simulink model "simulation_diffeomorfisme"  (R2020a)
settings: Solver=VariableStepAuto  StartTime=0.0  StopTime=100  RelTol=1e-3
values from neighbouring files (symbols this model uses):
  a = 1    [Adap.m]    (also in Adaptive_control_Non_linear.m = 2; HOSM.m; projet_AAV.m; sys.m)
  b = 2    [Adaptive_Control_Linear.m]    (also in Adaptive_control_Non_linear.m; HOSM.m = 1; feedback-integrator.m = 3; mini_projet.m = 3)
settings Model: Creator=lenovo  LastModifiedBy=lenovo

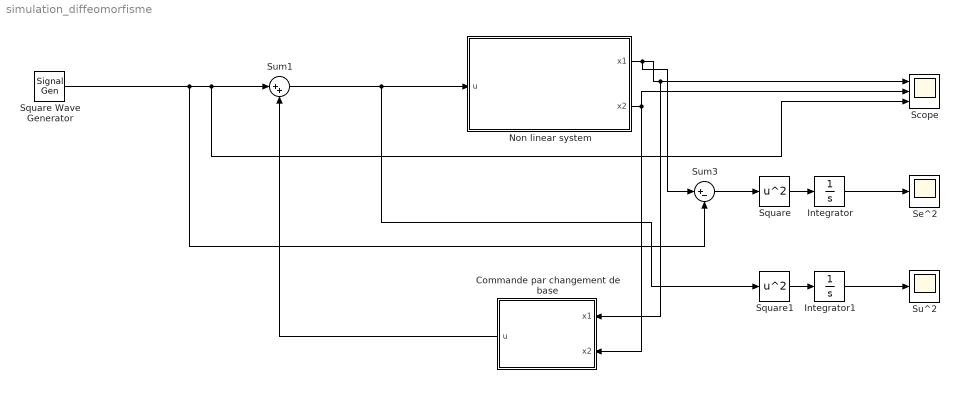
== system simulation_diffeomorfisme ==
  Commande par changement de base : Subsystem
  Integrator : Integrator
  Integrator1 : Integrator
  Non linear system : Subsystem
  Scope : Scope  NumInputPorts=3
  Se^2 : Scope
  Square : Math  Operator=square  SaturateOnIntegerOverflow=on
  Square Wave Generator : SignalGenerator  WaveForm=square  Frequency=0.1  Units=rad/sec
  Square1 : Math  Operator=square  SaturateOnIntegerOverflow=on
  Su^2 : Scope
  Sum1 : Sum  Inputs=|++
  Sum3 : Sum  Inputs=|+-
  wires:
  Non linear system/1(x1) -> Sum3/1, Commande par changement de base/1(x1), Scope/1
  Non linear system/2(x2) -> Commande par changement de base/2(x2), Scope/2
  Sum1/1 -> Square1/1, Non linear system/1(u)
  Commande par changement de base/1(u) -> Sum1/2
  Sum3/1 -> Square/1
  Square/1 -> Integrator/1
  Integrator/1 -> Se^2/1
  Integrator1/1 -> Su^2/1
  Square1/1 -> Integrator1/1
  Square Wave Generator/1 -> Sum3/2, Scope/3, Sum1/1

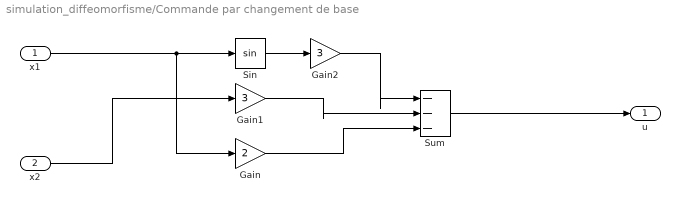
== system simulation_diffeomorfisme/Commande par changement de base ==
  x1 : Inport
  x2 : Inport  Port=2
  Gain : Gain  Gain=2
  Gain1 : Gain  Gain=3
  Gain2 : Gain  Gain=3
  Sin : Trigonometry
  Sum : Sum  Inputs=|---
  u : Outport
  wires:
  x1/1 -> Gain/1, Sin/1
  Sum/1 -> u/1
  Sin/1 -> Gain2/1
  x2/1 -> Gain1/1
  Gain2/1 -> Sum/1
  Gain1/1 -> Sum/2
  Gain/1 -> Sum/3

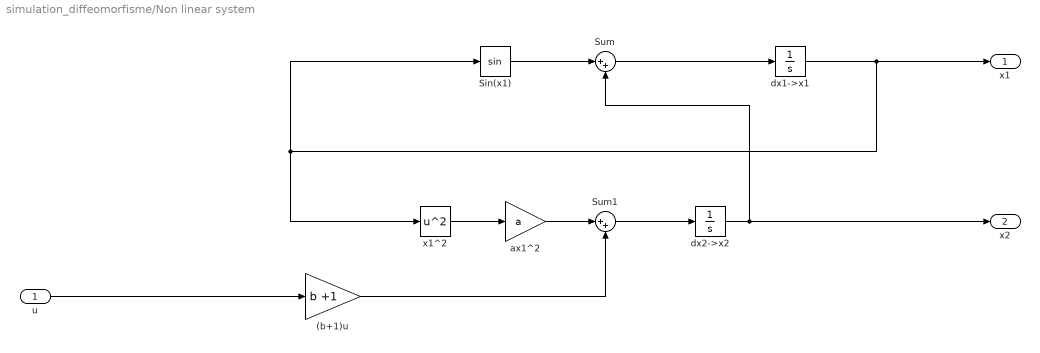
== system simulation_diffeomorfisme/Non linear system ==
  u : Inport
  (b+1)u : Gain  Gain=b +1
  Sin(x1) : Trigonometry
  Sum : Sum  Inputs=|++
  Sum1 : Sum  Inputs=|++
  ax1^2 : Gain  Gain=a
  dx1->x1 : Integrator
  dx2->x2 : Integrator
  x1^2 : Math  Operator=square  SaturateOnIntegerOverflow=on
  x1 : Outport
  x2 : Outport  Port=2
  wires:
  (b+1)u/1 -> Sum1/2
  dx2->x2/1 -> x2/1, Sum/2
  u/1 -> (b+1)u/1
  ax1^2/1 -> Sum1/1
  dx1->x1/1 -> Sin(x1)/1, x1^2/1, x1/1
  Sin(x1)/1 -> Sum/1
  x1^2/1 -> ax1^2/1
  Sum1/1 -> dx2->x2/1
  Sum/1 -> dx1->x1/1
